simulink model "blockdemo_sumofproducts"  (Simulink 7.6)
settings: Solver=ode45  StartTime=0.0  StopTime=10.0  RelTol=1e-3
InitFcn:
  | %% DSPBuilder Start
  | alt_dspbuilder_update_model(bdroot)
  | %% DSPBuilder End
libraries: allblocks_alteradspbuilder2 x18
settings Model: Creator=akarapet  LastModifiedBy=akarapet

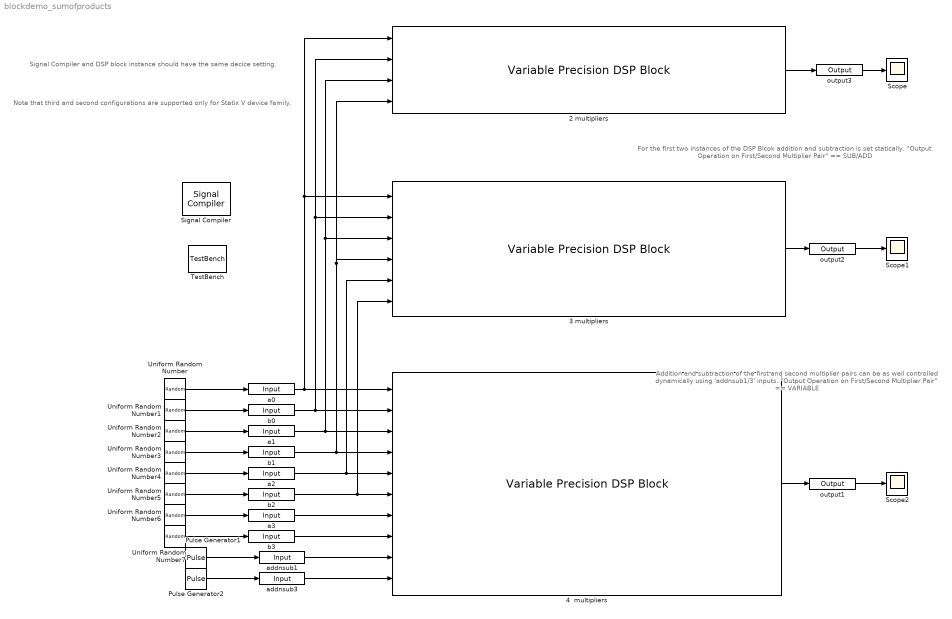
== system blockdemo_sumofproducts ==
  note: Addition and subtraction of the first and second multiplier pairs
      | can be as well controlled dynamically using 'addnsub1/3' inputs.
      |
      | "Output Operation on First/Second Multiplier Pair" == VARIABLE
  note: For the first two instances of the DSP Blcok addition and subtraction
      | is set statically.
      |
      | "Output Operation on First/Second Multiplier Pair" == SUB/ADD
  note: Signal Compiler and DSP block
      | instance should have the same
      | decice setting.
  note: Note that third and second
      | configurations are supported
      | only for Statix V device family.
  2 multipliers : allblocks_alteradspbuilder2/Variable Precision DSP Block  complex_model_delayed=0  model_delayed=0  device_family=Stratix V  used_mode_stratix=Other Modes  used_mode_arria=Other Modes  in_25x18_complex_mode=0  in_18x18plus36_mode=0  in_other_modes=1  number_of_mults=2  clock_ena_inputs=off  async_clear_inputs=off  bus_type=Signed Integer  bwl_A=16  bwr_A=0  width_A=16  chain_width=64  reg_inputs_A=on  A_inputs_reg_ena=ENABLE 0  bwl_B=16  bwr_B=0  width_B=16  reg_inputs_B=on  B_inputs_reg_ena=ENABLE 0  bwl_joint_A_B=8  bwr_joint_A_B=0  reg_joint_A_B_input=on  A_B_input_reg_ena=ENABLE 0  bwl_A_complex=8  bwr_A_complex=8  reg_complex_A=on  A_complex_inputs_reg_ena=ENABLE 0  bwl_B_complex=8  bwr_B_complex=8  reg_complex_B=on  B_complex_inputs_reg_ena=ENABLE 0  A_inputs_exist=1  B_inputs_exist=1  C_inputs_exist=0  coef_sel_inputs_exist=0  all_inputs_registered=1  no_input_registered=0  all_inputs_share_same_clocks=1  full_resolution=off  bwl_out=33  bwr_out=0  reg_output=off  output_reg_ena=ENABLE 0  systolic_regs_available=1  enable_systolic_regs=off  systolic_regs_used=0  basic_struct_ok_for_input_scan=1  input_scan_available=0  enable_input_scan=off  input_scan_used=0  input_scan_delay_regs_available=0  enable_input_scan_delay_regs=off  input_scan_delay_regs_used=0  basic_struct_ok_for_coef_rom=1  coef_rom_available=1  enable_coef_rom=off  coef_rom_used=0  basic_struct_ok_for_preadder=1  preadder_available=1  enable_preadder=off  preadder_used=0  preadder_direction=ADD  square_mode_available=0  enable_square_mode=off  square_mode_used=0  upper_limit_9bit=9  upper_limit_18bit=18  upper_limit_27bit=27  in_18x18_modes=1  in_27x27_modes=0  in_36x18_modes=0  in_36x36_mode=0  mult1_adder_available=1  mult1_direction=SUB  mult3_adder_available=0  mult3_direction=VARIABLE  chainout_adder_available=1  use_chainout_input=off  chainout_input_used=0  use_chainout_output=off  chainout_output_used=0  accum_available=1  enable_accum=off  accum_used=0  double_accum_available=0  enable_double_accum=off  double_accum_used=0  negate_available=1  mult_add_operation=ADD  rounding_constant_available=1  use_rounding_constant=off  rounding_constant_used=0  constant_value=1  bwl_C=8  bwr_C=0  bwl_coef=18  bwr_coef=0  mult0_coeffs=[0, 0, 0, 0, 0, 0, 0, 0]  mult1_coeffs=[0, 0, 0, 0, 0, 0, 0, 0]  mult2_coeffs=[0, 0, 0, 0, 0, 0, 0, 0]  mult3_coeffs=[0, 0, 0, 0, 0, 0, 0, 0]  reg_mult1_op_control=off  reg_mult3_op_control=on  reg_accum_control=off  reg_negate_control=off  control_regs_ena=ENABLE 0
  3 multipliers : allblocks_alteradspbuilder2/Variable Precision DSP Block  complex_model_delayed=0  model_delayed=0  device_family=Stratix V  used_mode_stratix=Other Modes  used_mode_arria=Other Modes  in_25x18_complex_mode=0  in_18x18plus36_mode=0  in_other_modes=1  number_of_mults=3  clock_ena_inputs=off  async_clear_inputs=off  bus_type=Signed Integer  bwl_A=16  bwr_A=0  width_A=16  chain_width=64  reg_inputs_A=on  A_inputs_reg_ena=ENABLE 0  bwl_B=16  bwr_B=0  width_B=16  reg_inputs_B=on  B_inputs_reg_ena=ENABLE 0  bwl_joint_A_B=8  bwr_joint_A_B=0  reg_joint_A_B_input=on  A_B_input_reg_ena=ENABLE 0  bwl_A_complex=8  bwr_A_complex=8  reg_complex_A=on  A_complex_inputs_reg_ena=ENABLE 0  bwl_B_complex=8  bwr_B_complex=8  reg_complex_B=on  B_complex_inputs_reg_ena=ENABLE 0  A_inputs_exist=1  B_inputs_exist=1  C_inputs_exist=0  coef_sel_inputs_exist=0  all_inputs_registered=1  no_input_registered=0  all_inputs_share_same_clocks=1  full_resolution=off  bwl_out=34  bwr_out=0  reg_output=on  output_reg_ena=ENABLE 0  systolic_regs_available=0  enable_systolic_regs=off  systolic_regs_used=0  basic_struct_ok_for_input_scan=1  input_scan_available=0  enable_input_scan=off  input_scan_used=0  input_scan_delay_regs_available=0  enable_input_scan_delay_regs=off  input_scan_delay_regs_used=0  basic_struct_ok_for_coef_rom=1  coef_rom_available=1  enable_coef_rom=off  coef_rom_used=0  basic_struct_ok_for_preadder=1  preadder_available=0  enable_preadder=off  preadder_used=0  preadder_direction=ADD  square_mode_available=0  enable_square_mode=off  square_mode_used=0  upper_limit_9bit=9  upper_limit_18bit=18  upper_limit_27bit=27  in_18x18_modes=1  in_27x27_modes=0  in_36x18_modes=0  in_36x36_mode=0  mult1_adder_available=1  mult1_direction=SUB  mult3_adder_available=0  mult3_direction=VARIABLE  chainout_adder_available=0  use_chainout_input=off  chainout_input_used=0  use_chainout_output=off  chainout_output_used=0  accum_available=0  enable_accum=off  accum_used=0  double_accum_available=0  enable_double_accum=off  double_accum_used=0  negate_available=0  mult_add_operation=ADD  rounding_constant_available=0  use_rounding_constant=off  rounding_constant_used=0  constant_value=1  bwl_C=8  bwr_C=0  bwl_coef=18  bwr_coef=0  mult0_coeffs=[0, 0, 0, 0, 0, 0, 0, 0]  mult1_coeffs=[0, 0, 0, 0, 0, 0, 0, 0]  mult2_coeffs=[0, 0, 0, 0, 0, 0, 0, 0]  mult3_coeffs=[0, 0, 0, 0, 0, 0, 0, 0]  reg_mult1_op_control=off  reg_mult3_op_control=on  reg_accum_control=off  reg_negate_control=off  control_regs_ena=ENABLE 0
  4  multipliers : allblocks_alteradspbuilder2/Variable Precision DSP Block  complex_model_delayed=0  model_delayed=0  device_family=Stratix V  used_mode_stratix=Other Modes  used_mode_arria=Other Modes  in_25x18_complex_mode=0  in_18x18plus36_mode=0  in_other_modes=1  number_of_mults=4  clock_ena_inputs=off  async_clear_inputs=off  bus_type=Signed Integer  bwl_A=16  bwr_A=0  width_A=16  chain_width=64  reg_inputs_A=on  A_inputs_reg_ena=ENABLE 0  bwl_B=16  bwr_B=0  width_B=16  reg_inputs_B=off  B_inputs_reg_ena=ENABLE 0  bwl_joint_A_B=8  bwr_joint_A_B=0  reg_joint_A_B_input=on  A_B_input_reg_ena=ENABLE 0  bwl_A_complex=8  bwr_A_complex=8  reg_complex_A=on  A_complex_inputs_reg_ena=ENABLE 0  bwl_B_complex=8  bwr_B_complex=8  reg_complex_B=on  B_complex_inputs_reg_ena=ENABLE 0  A_inputs_exist=1  B_inputs_exist=1  C_inputs_exist=0  coef_sel_inputs_exist=0  all_inputs_registered=0  no_input_registered=0  all_inputs_share_same_clocks=0  full_resolution=off  bwl_out=34  bwr_out=0  reg_output=on  output_reg_ena=ENABLE 0  systolic_regs_available=0  enable_systolic_regs=off  systolic_regs_used=0  basic_struct_ok_for_input_scan=1  input_scan_available=0  enable_input_scan=off  input_scan_used=0  input_scan_delay_regs_available=0  enable_input_scan_delay_regs=off  input_scan_delay_regs_used=0  basic_struct_ok_for_coef_rom=1  coef_rom_available=0  enable_coef_rom=off  coef_rom_used=0  basic_struct_ok_for_preadder=1  preadder_available=0  enable_preadder=off  preadder_used=0  preadder_direction=ADD  square_mode_available=0  enable_square_mode=off  square_mode_used=0  upper_limit_9bit=9  upper_limit_18bit=18  upper_limit_27bit=27  in_18x18_modes=1  in_27x27_modes=0  in_36x18_modes=0  in_36x36_mode=0  mult1_adder_available=1  mult1_direction=VARIABLE  mult3_adder_available=1  mult3_direction=VARIABLE  chainout_adder_available=0  use_chainout_input=off  chainout_input_used=0  use_chainout_output=off  chainout_output_used=0  accum_available=0  enable_accum=off  accum_used=0  double_accum_available=0  enable_double_accum=off  double_accum_used=0  negate_available=0  mult_add_operation=ADD  rounding_constant_available=0  use_rounding_constant=off  rounding_constant_used=0  constant_value=1  bwl_C=8  bwr_C=0  bwl_coef=18  bwr_coef=0  mult0_coeffs=[0, 0, 0, 0, 0, 0, 0, 0]  mult1_coeffs=[0, 0, 0, 0, 0, 0, 0, 0]  mult2_coeffs=[0, 0, 0, 0, 0, 0, 0, 0]  mult3_coeffs=[0, 0, 0, 0, 0, 0, 0, 0]  reg_mult1_op_control=off  reg_mult3_op_control=on  reg_accum_control=off  reg_negate_control=off  control_regs_ena=ENABLE 0
  Pulse Generator1 : DiscretePulseGenerator  Period=6  PulseWidth=3
  Pulse Generator2 : DiscretePulseGenerator  Period=5  PulseWidth=2
  Scope : Scope
  Scope1 : Scope
  Scope2 : Scope
      settings: SaveName=ScopeData2
  Signal Compiler : allblocks_alteradspbuilder2/Signal Compiler  DeviceFamily=Stratix V  DeviceName=AUTO  EnableSignalTap=off  SignalTapDepth=128  UseBoardBlock=off  StpUseDefaultClock=on  StpClock=Clock  ExportDir=<binary blob, 153 chars, not shown>
  TestBench : allblocks_alteradspbuilder2/TestBench  enable=on  advancedMode=off  modelSimGui=off  maxDisplayErrors=10  mismatchErrorLevel=Error  simdatafile=/data/akarapet/qshell_linux64_regtests/p4/dsp_builder/dsp_builder2/Documentation/DesignExamples/Tutorials/UnitBlocks/Arithmetic/VariablePrecisionDSPBlock/tb_blockdemo_sumofproducts/blockdemo_sumofproducts.simdata.tcl
  Uniform Random Number : UniformRandomNumber  Minimum=-128  Maximum=128  Seed=1231  SampleTime=1
  Uniform Random Number1 : UniformRandomNumber  Minimum=-128  Maximum=128  Seed=2365  SampleTime=1
  Uniform Random Number2 : UniformRandomNumber  Minimum=-128  Maximum=128  Seed=1234  SampleTime=1
  Uniform Random Number3 : UniformRandomNumber  Minimum=-128  Maximum=128  Seed=2365  SampleTime=1
  Uniform Random Number4 : UniformRandomNumber  Minimum=-128  Maximum=128  Seed=3451  SampleTime=1
  Uniform Random Number5 : UniformRandomNumber  Minimum=-128  Maximum=128  Seed=1111  SampleTime=1
  Uniform Random Number6 : UniformRandomNumber  Minimum=-128  Maximum=128  Seed=2333  SampleTime=1
  Uniform Random Number7 : UniformRandomNumber  Minimum=-128  Maximum=128  Seed=5111  SampleTime=1
  a0 : allblocks_alteradspbuilder2/Input  iofile=/data/akarapet/qshell_linux64_regtests/p4/dsp_builder/dsp_builder2/Documentation/DesignExamples/Tutorials/UnitBlocks/Arithmetic/VariablePrecisionDSPBlock/tb_blockdemo_sumofproducts/blockdemo%5Fsumofproducts_a0.salt  BusType=Signed Integer  bwl=16  bwr=0  SpecifyClock=off  clock=default_clock  PORTTYPE=Input  externalType=Inferred  allowFloatingPointOverride=on  logOutputs=off
  a1 : allblocks_alteradspbuilder2/Input  iofile=/data/akarapet/qshell_linux64_regtests/p4/dsp_builder/dsp_builder2/Documentation/DesignExamples/Tutorials/UnitBlocks/Arithmetic/VariablePrecisionDSPBlock/tb_blockdemo_sumofproducts/blockdemo%5Fsumofproducts_a1.salt  BusType=Signed Integer  bwl=16  bwr=0  SpecifyClock=off  clock=default_clock  PORTTYPE=Input  externalType=Inferred  allowFloatingPointOverride=on  logOutputs=off
  a2 : allblocks_alteradspbuilder2/Input  iofile=/data/akarapet/qshell_linux64_regtests/p4/dsp_builder/dsp_builder2/Documentation/DesignExamples/Tutorials/UnitBlocks/Arithmetic/VariablePrecisionDSPBlock/tb_blockdemo_sumofproducts/blockdemo%5Fsumofproducts_a2.salt  BusType=Signed Integer  bwl=16  bwr=0  SpecifyClock=off  clock=default_clock  PORTTYPE=Input  externalType=Inferred  allowFloatingPointOverride=on  logOutputs=off
  a3 : allblocks_alteradspbuilder2/Input  iofile=/data/akarapet/qshell_linux64_regtests/p4/dsp_builder/dsp_builder2/Documentation/DesignExamples/Tutorials/UnitBlocks/Arithmetic/VariablePrecisionDSPBlock/tb_blockdemo_sumofproducts/blockdemo%5Fsumofproducts_a3.salt  BusType=Signed Integer  bwl=16  bwr=0  SpecifyClock=off  clock=default_clock  PORTTYPE=Input  externalType=Inferred  allowFloatingPointOverride=on  logOutputs=off
  addnsub1 : allblocks_alteradspbuilder2/Input  iofile=/data/akarapet/qshell_linux64_regtests/p4/dsp_builder/dsp_builder2/Documentation/DesignExamples/Tutorials/UnitBlocks/Arithmetic/VariablePrecisionDSPBlock/tb_blockdemo_sumofproducts/blockdemo%5Fsumofproducts_addnsub1.salt  BusType=Single Bit  bwl=8  bwr=0  SpecifyClock=off  clock=default_clock  PORTTYPE=Input  externalType=Inferred  allowFloatingPointOverride=on  logOutputs=off
  addnsub3 : allblocks_alteradspbuilder2/Input  iofile=/data/akarapet/qshell_linux64_regtests/p4/dsp_builder/dsp_builder2/Documentation/DesignExamples/Tutorials/UnitBlocks/Arithmetic/VariablePrecisionDSPBlock/tb_blockdemo_sumofproducts/blockdemo%5Fsumofproducts_addnsub3.salt  BusType=Single Bit  bwl=8  bwr=0  SpecifyClock=off  clock=default_clock  PORTTYPE=Input  externalType=Inferred  allowFloatingPointOverride=on  logOutputs=off
  b0 : allblocks_alteradspbuilder2/Input  iofile=/data/akarapet/qshell_linux64_regtests/p4/dsp_builder/dsp_builder2/Documentation/DesignExamples/Tutorials/UnitBlocks/Arithmetic/VariablePrecisionDSPBlock/tb_blockdemo_sumofproducts/blockdemo%5Fsumofproducts_b0.salt  BusType=Signed Integer  bwl=16  bwr=0  SpecifyClock=off  clock=default_clock  PORTTYPE=Input  externalType=Inferred  allowFloatingPointOverride=on  logOutputs=off
  b1 : allblocks_alteradspbuilder2/Input  iofile=/data/akarapet/qshell_linux64_regtests/p4/dsp_builder/dsp_builder2/Documentation/DesignExamples/Tutorials/UnitBlocks/Arithmetic/VariablePrecisionDSPBlock/tb_blockdemo_sumofproducts/blockdemo%5Fsumofproducts_b1.salt  BusType=Signed Integer  bwl=16  bwr=0  SpecifyClock=off  clock=default_clock  PORTTYPE=Input  externalType=Inferred  allowFloatingPointOverride=on  logOutputs=off
  b2 : allblocks_alteradspbuilder2/Input  iofile=/data/akarapet/qshell_linux64_regtests/p4/dsp_builder/dsp_builder2/Documentation/DesignExamples/Tutorials/UnitBlocks/Arithmetic/VariablePrecisionDSPBlock/tb_blockdemo_sumofproducts/blockdemo%5Fsumofproducts_b2.salt  BusType=Signed Integer  bwl=16  bwr=0  SpecifyClock=off  clock=default_clock  PORTTYPE=Input  externalType=Inferred  allowFloatingPointOverride=on  logOutputs=off
  b3 : allblocks_alteradspbuilder2/Input  iofile=/data/akarapet/qshell_linux64_regtests/p4/dsp_builder/dsp_builder2/Documentation/DesignExamples/Tutorials/UnitBlocks/Arithmetic/VariablePrecisionDSPBlock/tb_blockdemo_sumofproducts/blockdemo%5Fsumofproducts_b3.salt  BusType=Signed Integer  bwl=16  bwr=0  SpecifyClock=off  clock=default_clock  PORTTYPE=Input  externalType=Inferred  allowFloatingPointOverride=on  logOutputs=off
  output1 : allblocks_alteradspbuilder2/Output  iofile=/data/akarapet/qshell_linux64_regtests/p4/dsp_builder/dsp_builder2/Documentation/DesignExamples/Tutorials/UnitBlocks/Arithmetic/VariablePrecisionDSPBlock/tb_blockdemo_sumofproducts/blockdemo%5Fsumofproducts_output1.capture  BusType=Signed Integer  bwl=34  bwr=0  externalType=Inferred  PORTTYPE=Output  allowFloatingPointOverride=on  logOutputs=off
  output2 : allblocks_alteradspbuilder2/Output  iofile=/data/akarapet/qshell_linux64_regtests/p4/dsp_builder/dsp_builder2/Documentation/DesignExamples/Tutorials/UnitBlocks/Arithmetic/VariablePrecisionDSPBlock/tb_blockdemo_sumofproducts/blockdemo%5Fsumofproducts_output2.capture  BusType=Signed Integer  bwl=34  bwr=0  externalType=Inferred  PORTTYPE=Output  allowFloatingPointOverride=on  logOutputs=off
  output3 : allblocks_alteradspbuilder2/Output  iofile=/data/akarapet/qshell_linux64_regtests/p4/dsp_builder/dsp_builder2/Documentation/DesignExamples/Tutorials/UnitBlocks/Arithmetic/VariablePrecisionDSPBlock/tb_blockdemo_sumofproducts/blockdemo%5Fsumofproducts_output3.capture  BusType=Signed Integer  bwl=32  bwr=0  externalType=Inferred  PORTTYPE=Output  allowFloatingPointOverride=on  logOutputs=off
  wires:
  Uniform Random Number/1 -> a0/1
  Uniform Random Number1/1 -> b0/1
  Uniform Random Number2/1 -> a1/1
  Uniform Random Number3/1 -> b1/1
  Uniform Random Number4/1 -> a2/1
  Uniform Random Number5/1 -> b2/1
  Uniform Random Number6/1 -> a3/1
  Uniform Random Number7/1 -> b3/1
  4  multipliers/1 -> output1/1
  a0/1 -> 4  multipliers/1, 3 multipliers/1, 2 multipliers/1
  b0/1 -> 4  multipliers/2, 3 multipliers/2, 2 multipliers/2
  a1/1 -> 4  multipliers/3, 3 multipliers/3, 2 multipliers/3
  b1/1 -> 4  multipliers/4, 3 multipliers/4, 2 multipliers/4
  a2/1 -> 4  multipliers/5, 3 multipliers/5
  b2/1 -> 4  multipliers/6, 3 multipliers/6
  a3/1 -> 4  multipliers/7
  b3/1 -> 4  multipliers/8
  addnsub1/1 -> 4  multipliers/9
  addnsub3/1 -> 4  multipliers/10
  Pulse Generator2/1 -> addnsub3/1
  Pulse Generator1/1 -> addnsub1/1
  3 multipliers/1 -> output2/1
  2 multipliers/1 -> output3/1
  output3/1 -> Scope/1
  output2/1 -> Scope1/1
  output1/1 -> Scope2/1
